simulink model "I2C_V2"  (R2017b)
settings: Solver=FixedStepAuto  StartTime=0.0  StopTime=10.0  RelTol=1e-3
PreLoadFcn:
  | waijung.modelPreload; % Required for working with Waijung Blockset. Do not remove.
undefined symbols (not defined in the file): HSEOSC, Link, LQFP100, ST, STM32F407VG
libraries: simulink x51, stm32f4_i2c_lib x7, stm32f4_io_lib x2, stm32f4_device_config_lib x1
(part 2 of 2)

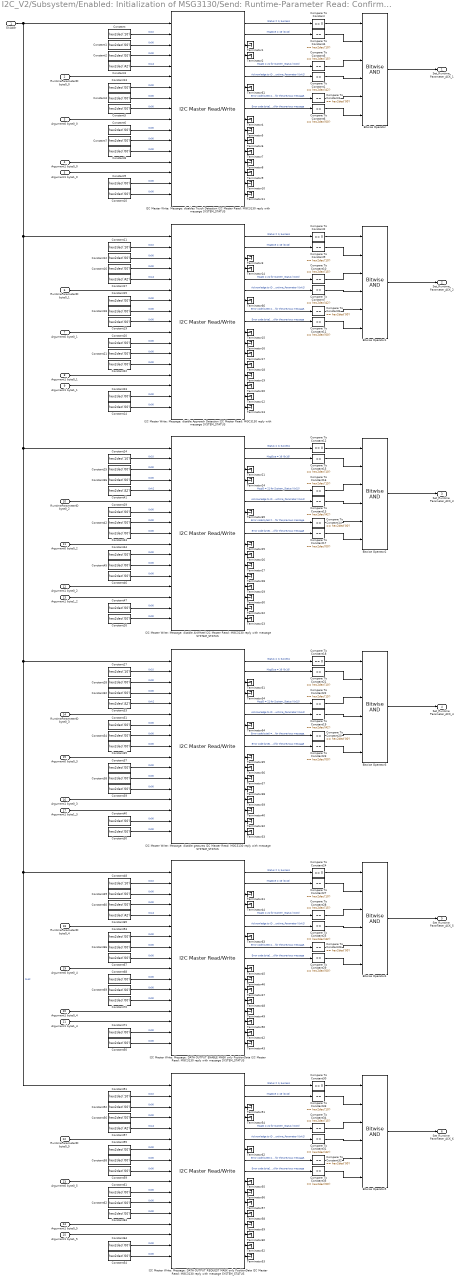
== system I2C_V2/Subsystem/Enabled: Initialization of MSG3130/Send: Runtime-Parameter Read: Confirmation Runtime-Parameter set ==
  SlvAddr : Inport
  RuntimeParameterID byte0_0 : Inport  Port=2
  Argument0 byte0_0 : Inport  Port=3
  Argument1 byte0_0 : Inport  Port=4
  Argument1 byte1_0 : Inport  Port=5
  RuntimeParameterID byte0_1 : Inport  Port=6
  Argument0 byte0_1 : Inport  Port=7
  Argument1 byte0_1 : Inport  Port=8
  Argument1 byte1_1 : Inport  Port=9
  RuntimeParameterID byte0_2 : Inport  Port=10
  Argument0 byte0_2 : Inport  Port=11
  Argument1 byte0_2 : Inport  Port=12
  Argument1 byte1_2 : Inport  Port=13
  RuntimeParameterID byte0_3 : Inport  Port=14
  Argument0 byte0_3 : Inport  Port=15
  Argument1 byte0_3 : Inport  Port=16
  Argument1 byte1_3 : Inport  Port=17
  RuntimeParameterID byte0_4 : Inport  Port=18
  Argument0 byte0_4 : Inport  Port=19
  Argument1 byte0_4 : Inport  Port=20
  Argument1 byte1_4 : Inport  Port=21
  RuntimeParameterID byte0_5 : Inport  Port=22
  Argument0 byte0_5 : Inport  Port=23
  Argument1 byte0_5 : Inport  Port=24
  Argument1 byte1_5 : Inport  Port=25
  Bitwise Operator{,1..5} (6 alike) : simulink/Logic and Bit Operations/Bitwise Operator  logicop=AND  UseBitMask=off  NumInputPorts=6  BitMask=bin2dec('11011001')  BitMaskRealWorld=Stored Integer
  Compare To Constant{,2,12,18,24,30} (6 alike) : simulink/Logic and Bit Operations/Compare To Constant  relop===  const=0  OutDataTypeStr=boolean  ZeroCross=off
  Compare To Constant{1,7,13,19,25,31} (6 alike) : simulink/Logic and Bit Operations/Compare To Constant  relop===  const=hex2dec('A2')  OutDataTypeStr=boolean  ZeroCross=off
  Compare To Constant{5,10,16,22,28,34} (6 alike) : simulink/Logic and Bit Operations/Compare To Constant  relop===  const=hex2dec('15')  OutDataTypeStr=boolean  ZeroCross=off
  Compare To Constant{3,6,8,11,14,17,20,23,26,29,32,35} (12 alike) : simulink/Logic and Bit Operations/Compare To Constant  relop===  const=hex2dec('00')  OutDataTypeStr=boolean  ZeroCross=off
  Compare To Constant{4,9,15,21,27,33} (6 alike) : simulink/Logic and Bit Operations/Compare To Constant  relop===  const=hex2dec('10')  OutDataTypeStr=boolean  ZeroCross=off
  Constant{,11,24,27,48,51} (6 alike) : Constant  Value=hex2dec('10')  OutDataTypeStr=uint8
  Constant{1..2,4..10,12..16,18..23,25..26,28..32,34..40,42..47,49..50,52..56,58..64,66..71} (60 alike) : Constant  Value=hex2dec('00')  OutDataTypeStr=uint8
  Constant{3,17,33,41,57,65} (6 alike) : Constant  Value=hex2dec('A2')  OutDataTypeStr=uint8
  I2C Master Write: Message: DATA OUTPUT ENABLE MASK only PositionData I2C Master Read: MGC3130 reply with message SYSTEM_STATUS : stm32f4_i2c_lib/I2C Master Read//Write  configuration=Transaction  module=1  lastmodule=3  transfer=Blocking  dutycycle=TLow/THigh = 2  clkspeed=400  timeout=25  writecount=16  readcount=16  sdapin=C9  sclpin=A8  waitwritetime=1  forcestop=on  inputtypearray=[17 3 3 3 3 3 3 3 3 3 3 3 3 3 3 3 3 3]  outputtypearray=[17 3 3 3 3 3 3 3 3 3 3 3 3 3 3 3 3 3]  confstr="[\"C\",\"9\",\"A\",\"8\",\"1\",\"1\",\"6\",\"0\",\"I2C_DutyCycle_2\",\"1\",\"on\"]"  sampletime=0.005  sampletimestr=-1  blockid=<binary blob, 200 chars, not shown>
  I2C Master Write: Message: DATA OUTPUT REQUEST MASK only PositionData I2C Master Read: MGC3130 reply with message SYSTEM_STATUS : stm32f4_i2c_lib/I2C Master Read//Write  configuration=Transaction  module=1  lastmodule=3  transfer=Blocking  dutycycle=TLow/THigh = 2  clkspeed=400  timeout=25  writecount=16  readcount=16  sdapin=C9  sclpin=A8  waitwritetime=1  forcestop=on  inputtypearray=[17 3 3 3 3 3 3 3 3 3 3 3 3 3 3 3 3 3]  outputtypearray=[17 3 3 3 3 3 3 3 3 3 3 3 3 3 3 3 3 3]  confstr="[\"C\",\"9\",\"A\",\"8\",\"1\",\"1\",\"6\",\"0\",\"I2C_DutyCycle_2\",\"1\",\"on\"]"  sampletime=0.005  sampletimestr=-1  blockid=<binary blob, 201 chars, not shown>
  "I2C Master Write: Message: disable AirWheel I2C Master Read: MGC3130 reply with message SYSTEM_STATUS " : stm32f4_i2c_lib/I2C Master Read//Write  configuration=Transaction  module=1  lastmodule=3  transfer=Blocking  dutycycle=TLow/THigh = 2  clkspeed=400  timeout=25  writecount=16  readcount=16  sdapin=C9  sclpin=A8  waitwritetime=1  forcestop=on  inputtypearray=[17 3 3 3 3 3 3 3 3 3 3 3 3 3 3 3 3 3]  outputtypearray=[17 3 3 3 3 3 3 3 3 3 3 3 3 3 3 3 3 3]  confstr="[\"C\",\"9\",\"A\",\"8\",\"1\",\"1\",\"6\",\"0\",\"I2C_DutyCycle_2\",\"1\",\"on\"]"  sampletime=0.005  sampletimestr=-1  blockid=<binary blob, 179 chars, not shown>
  "I2C Master Write: Message: disable Approach Detection I2C Master Read: MGC3130 reply with message SYSTEM_STATUS " : stm32f4_i2c_lib/I2C Master Read//Write  configuration=Transaction  module=1  lastmodule=3  transfer=Blocking  dutycycle=TLow/THigh = 2  clkspeed=400  timeout=25  writecount=16  readcount=16  sdapin=C9  sclpin=A8  waitwritetime=1  forcestop=on  inputtypearray=[17 3 3 3 3 3 3 3 3 3 3 3 3 3 3 3 3 3]  outputtypearray=[17 3 3 3 3 3 3 3 3 3 3 3 3 3 3 3 3 3]  confstr="[\"C\",\"9\",\"A\",\"8\",\"1\",\"1\",\"6\",\"0\",\"I2C_DutyCycle_2\",\"1\",\"on\"]"  sampletime=0.005  sampletimestr=-1  blockid=<binary blob, 188 chars, not shown>
  I2C Master Write: Message: disable gestures I2C Master Read: MGC3130 reply with message SYSTEM_STATUS : stm32f4_i2c_lib/I2C Master Read//Write  configuration=Transaction  module=1  lastmodule=3  transfer=Blocking  dutycycle=TLow/THigh = 2  clkspeed=400  timeout=25  writecount=16  readcount=16  sdapin=C9  sclpin=A8  waitwritetime=1  forcestop=on  inputtypearray=[17 3 3 3 3 3 3 3 3 3 3 3 3 3 3 3 3 3]  outputtypearray=[17 3 3 3 3 3 3 3 3 3 3 3 3 3 3 3 3 3]  confstr="[\"C\",\"9\",\"A\",\"8\",\"1\",\"1\",\"6\",\"0\",\"I2C_DutyCycle_2\",\"1\",\"on\"]"  sampletime=0.005  sampletimestr=-1  blockid=<binary blob, 179 chars, not shown>
  "I2C Master Write: Message: disables Touch Detection I2C Master Read: MGC3130 reply with message SYSTEM_STATUS " : stm32f4_i2c_lib/I2C Master Read//Write  configuration=Transaction  module=1  lastmodule=3  transfer=Blocking  dutycycle=TLow/THigh = 2  clkspeed=400  timeout=25  writecount=16  readcount=16  sdapin=C9  sclpin=A8  waitwritetime=1  forcestop=on  inputtypearray=[17 3 3 3 3 3 3 3 3 3 3 3 3 3 3 3 3 3]  outputtypearray=[17 3 3 3 3 3 3 3 3 3 3 3 3 3 3 3 3 3]  confstr="[\"C\",\"9\",\"A\",\"8\",\"1\",\"1\",\"6\",\"0\",\"I2C_DutyCycle_2\",\"1\",\"on\"]"  sampletime=0.005  sampletimestr=-1  blockid=<binary blob, 186 chars, not shown>
  Terminator{1..66} (66 alike) : Terminator
  Set_Runtime_Parameter_ACK_1 : Outport
  Set_Runtime_Parameter_ACK_2 : Outport  Port=2
  Set_Runtime_Parameter_ACK_3 : Outport  Port=3
  Set_Runtime_Parameter_ACK_4 : Outport  Port=4
  Set_Runtime_Parameter_ACK_5 : Outport  Port=5
  Set_Runtime_Parameter_ACK_6 : Outport  Port=6
  wires:
  "I2C Master Write: Message: disables Touch Detection I2C Master Read: MGC3130 reply with message SYSTEM_STATUS "/6 -> Compare To Constant1/1  "Acknowledge to ID 162, Set_Runtime_Parameter (0xA2)"
  Constant13/1 -> "I2C Master Write: Message: disables Touch Detection I2C Master Read: MGC3130 reply with message SYSTEM_STATUS "/7  "0x00"
  "I2C Master Write: Message: disables Touch Detection I2C Master Read: MGC3130 reply with message SYSTEM_STATUS "/17 -> Terminator11/1
  Constant9/1 -> "I2C Master Write: Message: disables Touch Detection I2C Master Read: MGC3130 reply with message SYSTEM_STATUS "/16  "0x00"
  "I2C Master Write: Message: disables Touch Detection I2C Master Read: MGC3130 reply with message SYSTEM_STATUS "/9 -> Compare To Constant6/1  "Error code byte1 = 0, for no Error returned for the previous message"
  Constant/1 -> "I2C Master Write: Message: disables Touch Detection I2C Master Read: MGC3130 reply with message SYSTEM_STATUS "/2  "0x10"
  Constant5/1 -> "I2C Master Write: Message: disables Touch Detection I2C Master Read: MGC3130 reply with message SYSTEM_STATUS "/9  "0x00"
  "I2C Master Write: Message: disables Touch Detection I2C Master Read: MGC3130 reply with message SYSTEM_STATUS "/2 -> Compare To Constant4/1  "MsgSize = 16 (0x10)"
  Constant3/1 -> "I2C Master Write: Message: disables Touch Detection I2C Master Read: MGC3130 reply with message SYSTEM_STATUS "/5  "0xA2"
  "I2C Master Write: Message: disables Touch Detection I2C Master Read: MGC3130 reply with message SYSTEM_STATUS "/12 -> Terminator6/1
  "I2C Master Write: Message: disables Touch Detection I2C Master Read: MGC3130 reply with message SYSTEM_STATUS "/4 -> Terminator2/1
  Constant4/1 -> "I2C Master Write: Message: disables Touch Detection I2C Master Read: MGC3130 reply with message SYSTEM_STATUS "/8  "0x00"
  Constant1/1 -> "I2C Master Write: Message: disables Touch Detection I2C Master Read: MGC3130 reply with message SYSTEM_STATUS "/3  "0x00"
  Constant2/1 -> "I2C Master Write: Message: disables Touch Detection I2C Master Read: MGC3130 reply with message SYSTEM_STATUS "/4  "0x00"
  "I2C Master Write: Message: disables Touch Detection I2C Master Read: MGC3130 reply with message SYSTEM_STATUS "/8 -> Compare To Constant3/1  "Error code byte0 = 0, for no Error returned for the previous message."
  "I2C Master Write: Message: disables Touch Detection I2C Master Read: MGC3130 reply with message SYSTEM_STATUS "/13 -> Terminator7/1
  Constant6/1 -> "I2C Master Write: Message: disables Touch Detection I2C Master Read: MGC3130 reply with message SYSTEM_STATUS "/11  "0x00"
  "I2C Master Write: Message: disables Touch Detection I2C Master Read: MGC3130 reply with message SYSTEM_STATUS "/10 -> Terminator4/1
  "I2C Master Write: Message: disables Touch Detection I2C Master Read: MGC3130 reply with message SYSTEM_STATUS "/15 -> Terminator9/1
  "I2C Master Write: Message: disables Touch Detection I2C Master Read: MGC3130 reply with message SYSTEM_STATUS "/5 -> Compare To Constant5/1  "MsgID = 21 for System_Status (0x15)"
  "I2C Master Write: Message: disables Touch Detection I2C Master Read: MGC3130 reply with message SYSTEM_STATUS "/14 -> Terminator8/1
  "I2C Master Write: Message: disables Touch Detection I2C Master Read: MGC3130 reply with message SYSTEM_STATUS "/3 -> Terminator1/1
  Constant8/1 -> "I2C Master Write: Message: disables Touch Detection I2C Master Read: MGC3130 reply with message SYSTEM_STATUS "/13  "0x00"
  Constant10/1 -> "I2C Master Write: Message: disables Touch Detection I2C Master Read: MGC3130 reply with message SYSTEM_STATUS "/17  "0x00"
  "I2C Master Write: Message: disables Touch Detection I2C Master Read: MGC3130 reply with message SYSTEM_STATUS "/1 -> Compare To Constant/1  "Status = 0, Success"
  "I2C Master Write: Message: disables Touch Detection I2C Master Read: MGC3130 reply with message SYSTEM_STATUS "/11 -> Terminator5/1
  Constant7/1 -> "I2C Master Write: Message: disables Touch Detection I2C Master Read: MGC3130 reply with message SYSTEM_STATUS "/12  "0x00"
  "I2C Master Write: Message: disables Touch Detection I2C Master Read: MGC3130 reply with message SYSTEM_STATUS "/16 -> Terminator10/1
  RuntimeParameterID byte0_0/1 -> "I2C Master Write: Message: disables Touch Detection I2C Master Read: MGC3130 reply with message SYSTEM_STATUS "/6
  Argument0 byte0_0/1 -> "I2C Master Write: Message: disables Touch Detection I2C Master Read: MGC3130 reply with message SYSTEM_STATUS "/10
  Argument1 byte0_0/1 -> "I2C Master Write: Message: disables Touch Detection I2C Master Read: MGC3130 reply with message SYSTEM_STATUS "/14
  Argument1 byte1_0/1 -> "I2C Master Write: Message: disables Touch Detection I2C Master Read: MGC3130 reply with message SYSTEM_STATUS "/15
  Constant11/1 -> "I2C Master Write: Message: disable Approach Detection I2C Master Read: MGC3130 reply with message SYSTEM_STATUS "/2  "0x10"
  Constant16/1 -> "I2C Master Write: Message: disable Approach Detection I2C Master Read: MGC3130 reply with message SYSTEM_STATUS "/4  "0x00"
  Constant17/1 -> "I2C Master Write: Message: disable Approach Detection I2C Master Read: MGC3130 reply with message SYSTEM_STATUS "/5  "0xA2"
  Constant23/1 -> "I2C Master Write: Message: disable Approach Detection I2C Master Read: MGC3130 reply with message SYSTEM_STATUS "/16  "0x00"
  Constant19/1 -> "I2C Master Write: Message: disable Approach Detection I2C Master Read: MGC3130 reply with message SYSTEM_STATUS "/9  "0x00"
  RuntimeParameterID byte0_1/1 -> "I2C Master Write: Message: disable Approach Detection I2C Master Read: MGC3130 reply with message SYSTEM_STATUS "/6
  Argument0 byte0_1/1 -> "I2C Master Write: Message: disable Approach Detection I2C Master Read: MGC3130 reply with message SYSTEM_STATUS "/10
  Argument1 byte1_1/1 -> "I2C Master Write: Message: disable Approach Detection I2C Master Read: MGC3130 reply with message SYSTEM_STATUS "/15
  Constant18/1 -> "I2C Master Write: Message: disable Approach Detection I2C Master Read: MGC3130 reply with message SYSTEM_STATUS "/8  "0x00"
  Argument1 byte0_1/1 -> "I2C Master Write: Message: disable Approach Detection I2C Master Read: MGC3130 reply with message SYSTEM_STATUS "/14
  Constant15/1 -> "I2C Master Write: Message: disable Approach Detection I2C Master Read: MGC3130 reply with message SYSTEM_STATUS "/7  "0x00"
  Constant22/1 -> "I2C Master Write: Message: disable Approach Detection I2C Master Read: MGC3130 reply with message SYSTEM_STATUS "/13  "0x00"
  Constant14/1 -> "I2C Master Write: Message: disable Approach Detection I2C Master Read: MGC3130 reply with message SYSTEM_STATUS "/17  "0x00"
  Constant12/1 -> "I2C Master Write: Message: disable Approach Detection I2C Master Read: MGC3130 reply with message SYSTEM_STATUS "/3  "0x00"
  Constant21/1 -> "I2C Master Write: Message: disable Approach Detection I2C Master Read: MGC3130 reply with message SYSTEM_STATUS "/12  "0x00"
  Constant20/1 -> "I2C Master Write: Message: disable Approach Detection I2C Master Read: MGC3130 reply with message SYSTEM_STATUS "/11  "0x00"
  Argument1 byte1_3/1 -> I2C Master Write: Message: disable gestures I2C Master Read: MGC3130 reply with message SYSTEM_STATUS/15
  Constant27/1 -> I2C Master Write: Message: disable gestures I2C Master Read: MGC3130 reply with message SYSTEM_STATUS/2  "0x10"
  Constant28/1 -> I2C Master Write: Message: disable gestures I2C Master Read: MGC3130 reply with message SYSTEM_STATUS/3  "0x00"
  Constant34/1 -> I2C Master Write: Message: disable gestures I2C Master Read: MGC3130 reply with message SYSTEM_STATUS/8  "0x00"
  Constant37/1 -> I2C Master Write: Message: disable gestures I2C Master Read: MGC3130 reply with message SYSTEM_STATUS/11  "0x00"
  RuntimeParameterID byte0_3/1 -> I2C Master Write: Message: disable gestures I2C Master Read: MGC3130 reply with message SYSTEM_STATUS/6
  Constant31/1 -> I2C Master Write: Message: disable gestures I2C Master Read: MGC3130 reply with message SYSTEM_STATUS/7  "0x00"
  Argument0 byte0_3/1 -> I2C Master Write: Message: disable gestures I2C Master Read: MGC3130 reply with message SYSTEM_STATUS/10
  Constant40/1 -> I2C Master Write: Message: disable gestures I2C Master Read: MGC3130 reply with message SYSTEM_STATUS/16  "0x00"
  Constant24/1 -> "I2C Master Write: Message: disable AirWheel I2C Master Read: MGC3130 reply with message SYSTEM_STATUS "/2  "0x10"
  Constant36/1 -> "I2C Master Write: Message: disable AirWheel I2C Master Read: MGC3130 reply with message SYSTEM_STATUS "/4  "0x00"
  Constant41/1 -> "I2C Master Write: Message: disable AirWheel I2C Master Read: MGC3130 reply with message SYSTEM_STATUS "/5  "0xA2"
  Constant47/1 -> "I2C Master Write: Message: disable AirWheel I2C Master Read: MGC3130 reply with message SYSTEM_STATUS "/16  "0x00"
  Constant35/1 -> I2C Master Write: Message: disable gestures I2C Master Read: MGC3130 reply with message SYSTEM_STATUS/9  "0x00"
  Constant43/1 -> "I2C Master Write: Message: disable AirWheel I2C Master Read: MGC3130 reply with message SYSTEM_STATUS "/9  "0x00"
  RuntimeParameterID byte0_2/1 -> "I2C Master Write: Message: disable AirWheel I2C Master Read: MGC3130 reply with message SYSTEM_STATUS "/6
  Argument0 byte0_2/1 -> "I2C Master Write: Message: disable AirWheel I2C Master Read: MGC3130 reply with message SYSTEM_STATUS "/10
  Argument1 byte0_3/1 -> I2C Master Write: Message: disable gestures I2C Master Read: MGC3130 reply with message SYSTEM_STATUS/14
  Argument1 byte1_2/1 -> "I2C Master Write: Message: disable AirWheel I2C Master Read: MGC3130 reply with message SYSTEM_STATUS "/15
  Constant42/1 -> "I2C Master Write: Message: disable AirWheel I2C Master Read: MGC3130 reply with message SYSTEM_STATUS "/8  "0x00"
  Constant38/1 -> I2C Master Write: Message: disable gestures I2C Master Read: MGC3130 reply with message SYSTEM_STATUS/12  "0x00"
  Constant29/1 -> "I2C Master Write: Message: disable AirWheel I2C Master Read: MGC3130 reply with message SYSTEM_STATUS "/7  "0x00"
  Argument1 byte0_2/1 -> "I2C Master Write: Message: disable AirWheel I2C Master Read: MGC3130 reply with message SYSTEM_STATUS "/14
  Constant46/1 -> "I2C Master Write: Message: disable AirWheel I2C Master Read: MGC3130 reply with message SYSTEM_STATUS "/13  "0x00"
  Constant32/1 -> I2C Master Write: Message: disable gestures I2C Master Read: MGC3130 reply with message SYSTEM_STATUS/4  "0x00"
  Constant30/1 -> I2C Master Write: Message: disable gestures I2C Master Read: MGC3130 reply with message SYSTEM_STATUS/17  "0x00"
  Constant26/1 -> "I2C Master Write: Message: disable AirWheel I2C Master Read: MGC3130 reply with message SYSTEM_STATUS "/17  "0x00"
  Constant25/1 -> "I2C Master Write: Message: disable AirWheel I2C Master Read: MGC3130 reply with message SYSTEM_STATUS "/3  "0x00"
  Constant39/1 -> I2C Master Write: Message: disable gestures I2C Master Read: MGC3130 reply with message SYSTEM_STATUS/13  "0x00"
  Constant33/1 -> I2C Master Write: Message: disable gestures I2C Master Read: MGC3130 reply with message SYSTEM_STATUS/5  "0xA2"
  Constant45/1 -> "I2C Master Write: Message: disable AirWheel I2C Master Read: MGC3130 reply with message SYSTEM_STATUS "/12  "0x00"
  Constant44/1 -> "I2C Master Write: Message: disable AirWheel I2C Master Read: MGC3130 reply with message SYSTEM_STATUS "/11  "0x00"
  Argument1 byte1_5/1 -> I2C Master Write: Message: DATA OUTPUT REQUEST MASK only PositionData I2C Master Read: MGC3130 reply with message SYSTEM_STATUS/15
  Constant51/1 -> I2C Master Write: Message: DATA OUTPUT REQUEST MASK only PositionData I2C Master Read: MGC3130 reply with message SYSTEM_STATUS/2  "0x10"
  Constant52/1 -> I2C Master Write: Message: DATA OUTPUT REQUEST MASK only PositionData I2C Master Read: MGC3130 reply with message SYSTEM_STATUS/3  "0x00"
  Constant58/1 -> I2C Master Write: Message: DATA OUTPUT REQUEST MASK only PositionData I2C Master Read: MGC3130 reply with message SYSTEM_STATUS/8  "0x00"
  Constant61/1 -> I2C Master Write: Message: DATA OUTPUT REQUEST MASK only PositionData I2C Master Read: MGC3130 reply with message SYSTEM_STATUS/11  "0x00"
  SlvAddr/1 -> "I2C Master Write: Message: disable Approach Detection I2C Master Read: MGC3130 reply with message SYSTEM_STATUS "/1, I2C Master Write: Message: DATA OUTPUT REQUEST MASK only PositionData I2C Master Read: MGC3130 reply with message SYSTEM_STATUS/1, I2C Master Write: Message: DATA OUTPUT ENABLE MASK only PositionData I2C Master Read: MGC3130 reply with message SYSTEM_STATUS/1, I2C Master Write: Message: disable gestures I2C Master Read: MGC3130 reply with message SYSTEM_STATUS/1, "I2C Master Write: Message: disable AirWheel I2C Master Read: MGC3130 reply with message SYSTEM_STATUS "/1, "I2C Master Write: Message: disables Touch Detection I2C Master Read: MGC3130 reply with message SYSTEM_STATUS "/1  "0x42"
  RuntimeParameterID byte0_5/1 -> I2C Master Write: Message: DATA OUTPUT REQUEST MASK only PositionData I2C Master Read: MGC3130 reply with message SYSTEM_STATUS/6
  Constant55/1 -> I2C Master Write: Message: DATA OUTPUT REQUEST MASK only PositionData I2C Master Read: MGC3130 reply with message SYSTEM_STATUS/7  "0x00"
  Argument0 byte0_5/1 -> I2C Master Write: Message: DATA OUTPUT REQUEST MASK only PositionData I2C Master Read: MGC3130 reply with message SYSTEM_STATUS/10
  Constant64/1 -> I2C Master Write: Message: DATA OUTPUT REQUEST MASK only PositionData I2C Master Read: MGC3130 reply with message SYSTEM_STATUS/16  "0x00"
  Constant48/1 -> I2C Master Write: Message: DATA OUTPUT ENABLE MASK only PositionData I2C Master Read: MGC3130 reply with message SYSTEM_STATUS/2  "0x10"
  Constant60/1 -> I2C Master Write: Message: DATA OUTPUT ENABLE MASK only PositionData I2C Master Read: MGC3130 reply with message SYSTEM_STATUS/4  "0x00"
  Constant65/1 -> I2C Master Write: Message: DATA OUTPUT ENABLE MASK only PositionData I2C Master Read: MGC3130 reply with message SYSTEM_STATUS/5  "0xA2"
  Constant71/1 -> I2C Master Write: Message: DATA OUTPUT ENABLE MASK only PositionData I2C Master Read: MGC3130 reply with message SYSTEM_STATUS/16  "0x00"
  Constant59/1 -> I2C Master Write: Message: DATA OUTPUT REQUEST MASK only PositionData I2C Master Read: MGC3130 reply with message SYSTEM_STATUS/9  "0x00"
  Constant67/1 -> I2C Master Write: Message: DATA OUTPUT ENABLE MASK only PositionData I2C Master Read: MGC3130 reply with message SYSTEM_STATUS/9  "0x00"
  RuntimeParameterID byte0_4/1 -> I2C Master Write: Message: DATA OUTPUT ENABLE MASK only PositionData I2C Master Read: MGC3130 reply with message SYSTEM_STATUS/6
  Argument0 byte0_4/1 -> I2C Master Write: Message: DATA OUTPUT ENABLE MASK only PositionData I2C Master Read: MGC3130 reply with message SYSTEM_STATUS/10
  Argument1 byte0_5/1 -> I2C Master Write: Message: DATA OUTPUT REQUEST MASK only PositionData I2C Master Read: MGC3130 reply with message SYSTEM_STATUS/14
  Argument1 byte1_4/1 -> I2C Master Write: Message: DATA OUTPUT ENABLE MASK only PositionData I2C Master Read: MGC3130 reply with message SYSTEM_STATUS/15
  Constant66/1 -> I2C Master Write: Message: DATA OUTPUT ENABLE MASK only PositionData I2C Master Read: MGC3130 reply with message SYSTEM_STATUS/8  "0x00"
  Constant62/1 -> I2C Master Write: Message: DATA OUTPUT REQUEST MASK only PositionData I2C Master Read: MGC3130 reply with message SYSTEM_STATUS/12  "0x00"
  Constant53/1 -> I2C Master Write: Message: DATA OUTPUT ENABLE MASK only PositionData I2C Master Read: MGC3130 reply with message SYSTEM_STATUS/7  "0x00"
  Argument1 byte0_4/1 -> I2C Master Write: Message: DATA OUTPUT ENABLE MASK only PositionData I2C Master Read: MGC3130 reply with message SYSTEM_STATUS/14
  Constant70/1 -> I2C Master Write: Message: DATA OUTPUT ENABLE MASK only PositionData I2C Master Read: MGC3130 reply with message SYSTEM_STATUS/13  "0x00"
  Constant56/1 -> I2C Master Write: Message: DATA OUTPUT REQUEST MASK only PositionData I2C Master Read: MGC3130 reply with message SYSTEM_STATUS/4  "0x00"
  Constant54/1 -> I2C Master Write: Message: DATA OUTPUT REQUEST MASK only PositionData I2C Master Read: MGC3130 reply with message SYSTEM_STATUS/17  "0x00"
  Constant50/1 -> I2C Master Write: Message: DATA OUTPUT ENABLE MASK only PositionData I2C Master Read: MGC3130 reply with message SYSTEM_STATUS/17  "0x00"
  Constant49/1 -> I2C Master Write: Message: DATA OUTPUT ENABLE MASK only PositionData I2C Master Read: MGC3130 reply with message SYSTEM_STATUS/3  "0x00"
  Constant63/1 -> I2C Master Write: Message: DATA OUTPUT REQUEST MASK only PositionData I2C Master Read: MGC3130 reply with message SYSTEM_STATUS/13  "0x00"
  Constant57/1 -> I2C Master Write: Message: DATA OUTPUT REQUEST MASK only PositionData I2C Master Read: MGC3130 reply with message SYSTEM_STATUS/5  "0xA2"
  Constant69/1 -> I2C Master Write: Message: DATA OUTPUT ENABLE MASK only PositionData I2C Master Read: MGC3130 reply with message SYSTEM_STATUS/12  "0x00"
  Constant68/1 -> I2C Master Write: Message: DATA OUTPUT ENABLE MASK only PositionData I2C Master Read: MGC3130 reply with message SYSTEM_STATUS/11  "0x00"
  "I2C Master Write: Message: disable Approach Detection I2C Master Read: MGC3130 reply with message SYSTEM_STATUS "/1 -> Compare To Constant2/1  "Status = 0, Success"
  "I2C Master Write: Message: disable Approach Detection I2C Master Read: MGC3130 reply with message SYSTEM_STATUS "/8 -> Compare To Constant8/1  "Error code byte0 = 0, for no Error returned for the previous message."
  "I2C Master Write: Message: disable Approach Detection I2C Master Read: MGC3130 reply with message SYSTEM_STATUS "/9 -> Compare To Constant11/1  "Error code byte1 = 0, for no Error returned for the previous message"
  "I2C Master Write: Message: disable Approach Detection I2C Master Read: MGC3130 reply with message SYSTEM_STATUS "/5 -> Compare To Constant10/1  "MsgID = 21 for System_Status (0x15)"
  "I2C Master Write: Message: disable Approach Detection I2C Master Read: MGC3130 reply with message SYSTEM_STATUS "/6 -> Compare To Constant7/1  "Acknowledge to ID 162, Set_Runtime_Parameter (0xA2)"
  "I2C Master Write: Message: disable Approach Detection I2C Master Read: MGC3130 reply with message SYSTEM_STATUS "/2 -> Compare To Constant9/1  "MsgSize = 16 (0x10)"
  "I2C Master Write: Message: disable Approach Detection I2C Master Read: MGC3130 reply with message SYSTEM_STATUS "/3 -> Terminator3/1
  "I2C Master Write: Message: disable Approach Detection I2C Master Read: MGC3130 reply with message SYSTEM_STATUS "/4 -> Terminator14/1
  "I2C Master Write: Message: disable Approach Detection I2C Master Read: MGC3130 reply with message SYSTEM_STATUS "/10 -> Terminator15/1
  "I2C Master Write: Message: disable Approach Detection I2C Master Read: MGC3130 reply with message SYSTEM_STATUS "/11 -> Terminator16/1
  "I2C Master Write: Message: disable Approach Detection I2C Master Read: MGC3130 reply with message SYSTEM_STATUS "/12 -> Terminator17/1
  "I2C Master Write: Message: disable Approach Detection I2C Master Read: MGC3130 reply with message SYSTEM_STATUS "/13 -> Terminator18/1
  "I2C Master Write: Message: disable Approach Detection I2C Master Read: MGC3130 reply with message SYSTEM_STATUS "/14 -> Terminator19/1
  "I2C Master Write: Message: disable Approach Detection I2C Master Read: MGC3130 reply with message SYSTEM_STATUS "/15 -> Terminator20/1
  "I2C Master Write: Message: disable Approach Detection I2C Master Read: MGC3130 reply with message SYSTEM_STATUS "/16 -> Terminator12/1
  "I2C Master Write: Message: disable Approach Detection I2C Master Read: MGC3130 reply with message SYSTEM_STATUS "/17 -> Terminator13/1
  "I2C Master Write: Message: disable AirWheel I2C Master Read: MGC3130 reply with message SYSTEM_STATUS "/1 -> Compare To Constant12/1  "Status = 0, Success"
  "I2C Master Write: Message: disable AirWheel I2C Master Read: MGC3130 reply with message SYSTEM_STATUS "/8 -> Compare To Constant14/1  "Error code byte0 = 0, for no Error returned for the previous message."
  "I2C Master Write: Message: disable AirWheel I2C Master Read: MGC3130 reply with message SYSTEM_STATUS "/9 -> Compare To Constant17/1  "Error code byte1 = 0, for no Error returned for the previous message"
  "I2C Master Write: Message: disable AirWheel I2C Master Read: MGC3130 reply with message SYSTEM_STATUS "/5 -> Compare To Constant16/1  "MsgID = 21 for System_Status (0x15)"
  "I2C Master Write: Message: disable AirWheel I2C Master Read: MGC3130 reply with message SYSTEM_STATUS "/6 -> Compare To Constant13/1  "Acknowledge to ID 162, Set_Runtime_Parameter (0xA2)"
  "I2C Master Write: Message: disable AirWheel I2C Master Read: MGC3130 reply with message SYSTEM_STATUS "/2 -> Compare To Constant15/1  "MsgSize = 16 (0x10)"
  I2C Master Write: Message: disable gestures I2C Master Read: MGC3130 reply with message SYSTEM_STATUS/1 -> Compare To Constant18/1  "Status = 0, Success"
  I2C Master Write: Message: disable gestures I2C Master Read: MGC3130 reply with message SYSTEM_STATUS/8 -> Compare To Constant20/1  "Error code byte0 = 0, for no Error returned for the previous message."
  I2C Master Write: Message: disable gestures I2C Master Read: MGC3130 reply with message SYSTEM_STATUS/9 -> Compare To Constant23/1  "Error code byte1 = 0, for no Error returned for the previous message"
  I2C Master Write: Message: disable gestures I2C Master Read: MGC3130 reply with message SYSTEM_STATUS/5 -> Compare To Constant22/1  "MsgID = 21 for System_Status (0x15)"
  I2C Master Write: Message: disable gestures I2C Master Read: MGC3130 reply with message SYSTEM_STATUS/6 -> Compare To Constant19/1  "Acknowledge to ID 162, Set_Runtime_Parameter (0xA2)"
  I2C Master Write: Message: disable gestures I2C Master Read: MGC3130 reply with message SYSTEM_STATUS/2 -> Compare To Constant21/1  "MsgSize = 16 (0x10)"
  I2C Master Write: Message: disable gestures I2C Master Read: MGC3130 reply with message SYSTEM_STATUS/17 -> Terminator33/1
  I2C Master Write: Message: DATA OUTPUT ENABLE MASK only PositionData I2C Master Read: MGC3130 reply with message SYSTEM_STATUS/1 -> Compare To Constant24/1  "Status = 0, Success"
  I2C Master Write: Message: DATA OUTPUT ENABLE MASK only PositionData I2C Master Read: MGC3130 reply with message SYSTEM_STATUS/8 -> Compare To Constant26/1  "Error code byte0 = 0, for no Error returned for the previous message."
  I2C Master Write: Message: DATA OUTPUT ENABLE MASK only PositionData I2C Master Read: MGC3130 reply with message SYSTEM_STATUS/9 -> Compare To Constant29/1  "Error code byte1 = 0, for no Error returned for the previous message"
  I2C Master Write: Message: DATA OUTPUT ENABLE MASK only PositionData I2C Master Read: MGC3130 reply with message SYSTEM_STATUS/5 -> Compare To Constant28/1  "MsgID = 21 for System_Status (0x15)"
  I2C Master Write: Message: DATA OUTPUT ENABLE MASK only PositionData I2C Master Read: MGC3130 reply with message SYSTEM_STATUS/6 -> Compare To Constant25/1  "Acknowledge to ID 162, Set_Runtime_Parameter (0xA2)"
  I2C Master Write: Message: DATA OUTPUT ENABLE MASK only PositionData I2C Master Read: MGC3130 reply with message SYSTEM_STATUS/2 -> Compare To Constant27/1  "MsgSize = 16 (0x10)"
  I2C Master Write: Message: DATA OUTPUT REQUEST MASK only PositionData I2C Master Read: MGC3130 reply with message SYSTEM_STATUS/1 -> Compare To Constant30/1  "Status = 0, Success"
  I2C Master Write: Message: DATA OUTPUT REQUEST MASK only PositionData I2C Master Read: MGC3130 reply with message SYSTEM_STATUS/8 -> Compare To Constant32/1  "Error code byte0 = 0, for no Error returned for the previous message."
  I2C Master Write: Message: DATA OUTPUT REQUEST MASK only PositionData I2C Master Read: MGC3130 reply with message SYSTEM_STATUS/9 -> Compare To Constant35/1  "Error code byte1 = 0, for no Error returned for the previous message"
  I2C Master Write: Message: DATA OUTPUT REQUEST MASK only PositionData I2C Master Read: MGC3130 reply with message SYSTEM_STATUS/5 -> Compare To Constant34/1  "MsgID = 21 for System_Status (0x15)"
  I2C Master Write: Message: DATA OUTPUT REQUEST MASK only PositionData I2C Master Read: MGC3130 reply with message SYSTEM_STATUS/6 -> Compare To Constant31/1  "Acknowledge to ID 162, Set_Runtime_Parameter (0xA2)"
  I2C Master Write: Message: DATA OUTPUT REQUEST MASK only PositionData I2C Master Read: MGC3130 reply with message SYSTEM_STATUS/2 -> Compare To Constant33/1  "MsgSize = 16 (0x10)"
  "I2C Master Write: Message: disable AirWheel I2C Master Read: MGC3130 reply with message SYSTEM_STATUS "/3 -> Terminator21/1
  "I2C Master Write: Message: disable AirWheel I2C Master Read: MGC3130 reply with message SYSTEM_STATUS "/4 -> Terminator24/1
  "I2C Master Write: Message: disable AirWheel I2C Master Read: MGC3130 reply with message SYSTEM_STATUS "/10 -> Terminator25/1
  "I2C Master Write: Message: disable AirWheel I2C Master Read: MGC3130 reply with message SYSTEM_STATUS "/11 -> Terminator26/1
  "I2C Master Write: Message: disable AirWheel I2C Master Read: MGC3130 reply with message SYSTEM_STATUS "/12 -> Terminator27/1
  "I2C Master Write: Message: disable AirWheel I2C Master Read: MGC3130 reply with message SYSTEM_STATUS "/13 -> Terminator28/1
  "I2C Master Write: Message: disable AirWheel I2C Master Read: MGC3130 reply with message SYSTEM_STATUS "/14 -> Terminator29/1
  "I2C Master Write: Message: disable AirWheel I2C Master Read: MGC3130 reply with message SYSTEM_STATUS "/15 -> Terminator30/1
  "I2C Master Write: Message: disable AirWheel I2C Master Read: MGC3130 reply with message SYSTEM_STATUS "/16 -> Terminator22/1
  "I2C Master Write: Message: disable AirWheel I2C Master Read: MGC3130 reply with message SYSTEM_STATUS "/17 -> Terminator23/1
  I2C Master Write: Message: disable gestures I2C Master Read: MGC3130 reply with message SYSTEM_STATUS/3 -> Terminator31/1
  I2C Master Write: Message: disable gestures I2C Master Read: MGC3130 reply with message SYSTEM_STATUS/4 -> Terminator34/1
  I2C Master Write: Message: disable gestures I2C Master Read: MGC3130 reply with message SYSTEM_STATUS/10 -> Terminator35/1
  I2C Master Write: Message: disable gestures I2C Master Read: MGC3130 reply with message SYSTEM_STATUS/11 -> Terminator36/1
  I2C Master Write: Message: disable gestures I2C Master Read: MGC3130 reply with message SYSTEM_STATUS/12 -> Terminator37/1
  I2C Master Write: Message: disable gestures I2C Master Read: MGC3130 reply with message SYSTEM_STATUS/13 -> Terminator38/1
  I2C Master Write: Message: disable gestures I2C Master Read: MGC3130 reply with message SYSTEM_STATUS/14 -> Terminator39/1
  I2C Master Write: Message: disable gestures I2C Master Read: MGC3130 reply with message SYSTEM_STATUS/15 -> Terminator40/1
  I2C Master Write: Message: disable gestures I2C Master Read: MGC3130 reply with message SYSTEM_STATUS/16 -> Terminator32/1
  I2C Master Write: Message: DATA OUTPUT ENABLE MASK only PositionData I2C Master Read: MGC3130 reply with message SYSTEM_STATUS/3 -> Terminator41/1
  I2C Master Write: Message: DATA OUTPUT ENABLE MASK only PositionData I2C Master Read: MGC3130 reply with message SYSTEM_STATUS/4 -> Terminator44/1
  I2C Master Write: Message: DATA OUTPUT ENABLE MASK only PositionData I2C Master Read: MGC3130 reply with message SYSTEM_STATUS/10 -> Terminator45/1
  I2C Master Write: Message: DATA OUTPUT ENABLE MASK only PositionData I2C Master Read: MGC3130 reply with message SYSTEM_STATUS/11 -> Terminator46/1
  I2C Master Write: Message: DATA OUTPUT ENABLE MASK only PositionData I2C Master Read: MGC3130 reply with message SYSTEM_STATUS/12 -> Terminator47/1
  I2C Master Write: Message: DATA OUTPUT ENABLE MASK only PositionData I2C Master Read: MGC3130 reply with message SYSTEM_STATUS/13 -> Terminator48/1
  I2C Master Write: Message: DATA OUTPUT ENABLE MASK only PositionData I2C Master Read: MGC3130 reply with message SYSTEM_STATUS/14 -> Terminator49/1
  I2C Master Write: Message: DATA OUTPUT ENABLE MASK only PositionData I2C Master Read: MGC3130 reply with message SYSTEM_STATUS/15 -> Terminator50/1
  I2C Master Write: Message: DATA OUTPUT ENABLE MASK only PositionData I2C Master Read: MGC3130 reply with message SYSTEM_STATUS/16 -> Terminator42/1
  I2C Master Write: Message: DATA OUTPUT ENABLE MASK only PositionData I2C Master Read: MGC3130 reply with message SYSTEM_STATUS/17 -> Terminator43/1
  I2C Master Write: Message: DATA OUTPUT REQUEST MASK only PositionData I2C Master Read: MGC3130 reply with message SYSTEM_STATUS/3 -> Terminator51/1
  I2C Master Write: Message: DATA OUTPUT REQUEST MASK only PositionData I2C Master Read: MGC3130 reply with message SYSTEM_STATUS/4 -> Terminator54/1
  I2C Master Write: Message: DATA OUTPUT REQUEST MASK only PositionData I2C Master Read: MGC3130 reply with message SYSTEM_STATUS/10 -> Terminator55/1
  I2C Master Write: Message: DATA OUTPUT REQUEST MASK only PositionData I2C Master Read: MGC3130 reply with message SYSTEM_STATUS/11 -> Terminator56/1
  I2C Master Write: Message: DATA OUTPUT REQUEST MASK only PositionData I2C Master Read: MGC3130 reply with message SYSTEM_STATUS/12 -> Terminator57/1
  I2C Master Write: Message: DATA OUTPUT REQUEST MASK only PositionData I2C Master Read: MGC3130 reply with message SYSTEM_STATUS/13 -> Terminator58/1
  I2C Master Write: Message: DATA OUTPUT REQUEST MASK only PositionData I2C Master Read: MGC3130 reply with message SYSTEM_STATUS/14 -> Terminator59/1
  I2C Master Write: Message: DATA OUTPUT REQUEST MASK only PositionData I2C Master Read: MGC3130 reply with message SYSTEM_STATUS/15 -> Terminator60/1
  I2C Master Write: Message: DATA OUTPUT REQUEST MASK only PositionData I2C Master Read: MGC3130 reply with message SYSTEM_STATUS/16 -> Terminator52/1
  I2C Master Write: Message: DATA OUTPUT REQUEST MASK only PositionData I2C Master Read: MGC3130 reply with message SYSTEM_STATUS/17 -> Terminator53/1
  Compare To Constant/1 -> Bitwise Operator/1
  Compare To Constant4/1 -> Bitwise Operator/2
  Compare To Constant5/1 -> Bitwise Operator/3
  Compare To Constant1/1 -> Bitwise Operator/4
  Bitwise Operator/1 -> Set_Runtime_Parameter_ACK_1/1
  Compare To Constant3/1 -> Bitwise Operator/5
  Compare To Constant6/1 -> Bitwise Operator/6
  "I2C Master Write: Message: disables Touch Detection I2C Master Read: MGC3130 reply with message SYSTEM_STATUS "/7 -> Terminator61/1
  Compare To Constant11/1 -> Bitwise Operator1/6
  Compare To Constant10/1 -> Bitwise Operator1/3
  Compare To Constant9/1 -> Bitwise Operator1/2
  Compare To Constant8/1 -> Bitwise Operator1/5
  Compare To Constant2/1 -> Bitwise Operator1/1
  Compare To Constant7/1 -> Bitwise Operator1/4
  Bitwise Operator1/1 -> Set_Runtime_Parameter_ACK_2/1
  Compare To Constant17/1 -> Bitwise Operator2/6
  Compare To Constant16/1 -> Bitwise Operator2/3
  Compare To Constant15/1 -> Bitwise Operator2/2
  Compare To Constant14/1 -> Bitwise Operator2/5
  Compare To Constant12/1 -> Bitwise Operator2/1
  Compare To Constant13/1 -> Bitwise Operator2/4
  Bitwise Operator2/1 -> Set_Runtime_Parameter_ACK_3/1
  Compare To Constant23/1 -> Bitwise Operator3/6
  Compare To Constant22/1 -> Bitwise Operator3/3
  Compare To Constant21/1 -> Bitwise Operator3/2
  Compare To Constant20/1 -> Bitwise Operator3/5
  Compare To Constant18/1 -> Bitwise Operator3/1
  Compare To Constant19/1 -> Bitwise Operator3/4
  Bitwise Operator3/1 -> Set_Runtime_Parameter_ACK_4/1
  Compare To Constant29/1 -> Bitwise Operator4/6
  Compare To Constant28/1 -> Bitwise Operator4/3
  Compare To Constant27/1 -> Bitwise Operator4/2
  Compare To Constant26/1 -> Bitwise Operator4/5
  Compare To Constant24/1 -> Bitwise Operator4/1
  Compare To Constant25/1 -> Bitwise Operator4/4
  Bitwise Operator4/1 -> Set_Runtime_Parameter_ACK_5/1
  Compare To Constant35/1 -> Bitwise Operator5/6
  Compare To Constant34/1 -> Bitwise Operator5/3
  Compare To Constant33/1 -> Bitwise Operator5/2
  Compare To Constant32/1 -> Bitwise Operator5/5
  Compare To Constant30/1 -> Bitwise Operator5/1
  Compare To Constant31/1 -> Bitwise Operator5/4
  Bitwise Operator5/1 -> Set_Runtime_Parameter_ACK_6/1
  I2C Master Write: Message: DATA OUTPUT REQUEST MASK only PositionData I2C Master Read: MGC3130 reply with message SYSTEM_STATUS/7 -> Terminator62/1
  I2C Master Write: Message: DATA OUTPUT ENABLE MASK only PositionData I2C Master Read: MGC3130 reply with message SYSTEM_STATUS/7 -> Terminator63/1
  I2C Master Write: Message: disable gestures I2C Master Read: MGC3130 reply with message SYSTEM_STATUS/7 -> Terminator64/1
  "I2C Master Write: Message: disable AirWheel I2C Master Read: MGC3130 reply with message SYSTEM_STATUS "/7 -> Terminator65/1
  "I2C Master Write: Message: disable Approach Detection I2C Master Read: MGC3130 reply with message SYSTEM_STATUS "/7 -> Terminator66/1
